simulink model "LevitadorMagnetico_ordenado"  (R2021a)
settings: Solver=ode1  StartTime=0.0  StopTime=1  FixedStep=0.001  RelTol=1e-3
settings Model: Creator=zeta  LastModifiedBy=valen

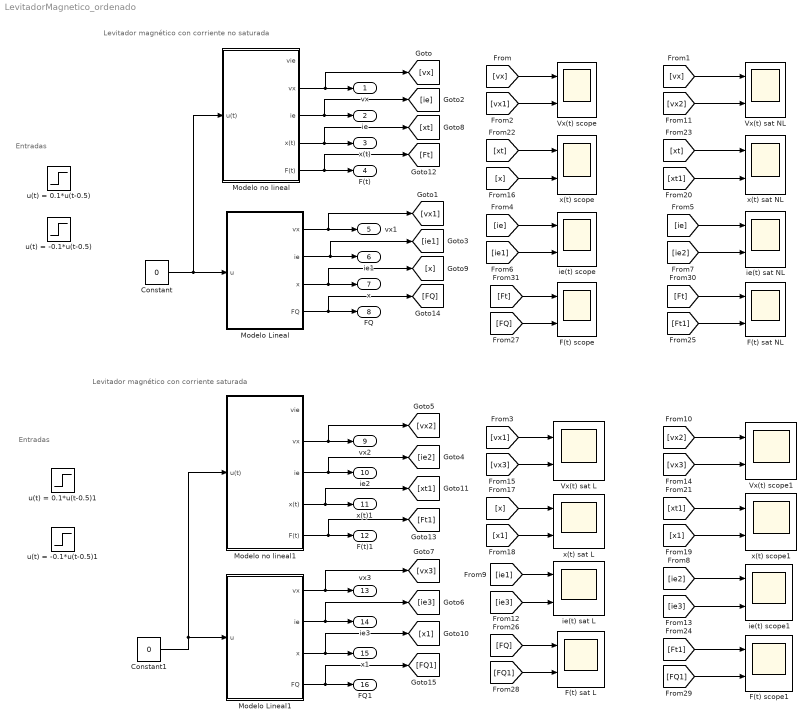
== system LevitadorMagnetico_ordenado ==
  note: Entradas
  note: Levitador magnético con corriente no saturada
  note: Levitador magnético con corriente saturada
  note: Entradas
  Constant : Constant  Value=0
  Constant1 : Constant  Value=0
  F(t) sat L : Scope  NumInputPorts=2
  F(t) sat NL : Scope  NumInputPorts=2
  F(t) scope : Scope  NumInputPorts=2
  F(t) scope1 : Scope  NumInputPorts=2
  Modelo Lineal : Subsystem  mask{Ka=3, Km=1, K1=5888, K2=1536, R=20, L=0.2, uQ=0, xQ=3.2, vxQ=-6.8, ieQ=0, vx_sat_sup=6.8, vx_sat_inf=-10+6.8, x_sat_sup=10-3.2, x_sat_inf=-3.2, m=0.15, g=1000}
      mask prompts: vx_sat_sup "(vx_sat_sup - vxQ)"; vx_sat_inf "(vx_sat_inf- vxQ)"; x_sat_sup "(x_sat_sup - xQ)"; x_sat_inf "(x_sat_inf  - xQ)"
      mask DialogControl Control2 Prompt: Punto de operación:
      mask DialogControl Control3 Prompt: Saturación:
      mask DialogControl Control4 Prompt: otros
  Modelo Lineal1 : Subsystem  mask{Ka=3, Km=1, K1=5888, K2=1536, R=20, L=0.2, uQ=0, xQ=3.2, vxQ=-6.8, ieQ=0, vx_sat_sup=6.8, vx_sat_inf=-10+6.8, x_sat_sup=10-3.2, x_sat_inf=-3.2, m=0.15, g=1000}
      mask prompts: vx_sat_sup "(vx_sat_sup - vxQ)"; vx_sat_inf "(vx_sat_inf- vxQ)"; x_sat_sup "(x_sat_sup - xQ)"; x_sat_inf "(x_sat_inf  - xQ)"
      mask DialogControl Control2 Prompt: Punto de operación:
      mask DialogControl Control3 Prompt: Saturación:
      mask DialogControl Control4 Prompt: otros
  Modelo no lineal : Subsystem
  Modelo no lineal1 : Subsystem
  Vx(t) sat L : Scope  NumInputPorts=2
  Vx(t) sat NL : Scope  NumInputPorts=2
  Vx(t) scope : Scope  NumInputPorts=2
  Vx(t) scope1 : Scope  NumInputPorts=2
  ie(t) sat L : Scope  NumInputPorts=2
  ie(t) sat NL : Scope  NumInputPorts=2
  ie(t) scope : Scope  NumInputPorts=2
  ie(t) scope1 : Scope  NumInputPorts=2
  u(t) = -0.1*u(t-0.5) : Step  Time=0.5  After=-0.1  SampleTime=0
  u(t) = -0.1*u(t-0.5)1 : Step  Time=0.5  After=-0.1  SampleTime=0
  u(t) = 0.1*u(t-0.5) : Step  Time=0.5  After=0.1  SampleTime=0
  u(t) = 0.1*u(t-0.5)1 : Step  Time=0.5  After=0.1  SampleTime=0
  x(t) sat L : Scope  NumInputPorts=2
  x(t) sat NL : Scope  NumInputPorts=2
  x(t) scope : Scope  NumInputPorts=2
  x(t) scope1 : Scope  NumInputPorts=2
  vx : Outport
  ie : Outport  Port=2
  x(t) : Outport  Port=3
  F(t) : Outport  Port=4
  vx1 : Outport  Port=5
  ie1 : Outport  Port=6
  x : Outport  Port=7
  FQ : Outport  Port=8
  vx2 : Outport  Port=9
  ie2 : Outport  Port=10
  x(t)1 : Outport  Port=11
  F(t)1 : Outport  Port=12
  vx3 : Outport  Port=13
  ie3 : Outport  Port=14
  x1 : Outport  Port=15
  FQ1 : Outport  Port=16
  wires:
  Modelo no lineal/2(vx) -> vx/1, [vx]
  Modelo no lineal/4(x(t)) -> x(t)/1, [xt]
  Modelo no lineal/5(F(t)) -> [Ft], F(t)/1
  Modelo Lineal/4(FQ) -> [FQ], FQ/1
  Modelo Lineal/2(ie) -> [ie1], ie1/1
  Modelo Lineal/1(vx) -> vx1/1, [vx1]
  Modelo Lineal/3(x) -> x/1, [x]
  Modelo no lineal/3(ie) -> ie/1, [ie]
  Constant/1 -> Modelo no lineal/1(u(t)), Modelo Lineal/1(u)
  Modelo Lineal1/4(FQ) -> FQ1/1, [FQ1]
  Modelo no lineal1/2(vx) -> vx2/1, [vx2]
  Modelo no lineal1/3(ie) -> ie2/1, [ie2]
  Constant1/1 -> Modelo no lineal1/1(u(t)), Modelo Lineal1/1(u)
  Modelo Lineal1/3(x) -> [x1], x1/1
  Modelo no lineal1/5(F(t)) -> [Ft1], F(t)1/1
  Modelo no lineal1/4(x(t)) -> [xt1], x(t)1/1
  Modelo Lineal1/2(ie) -> ie3/1, [ie3]
  Modelo Lineal1/1(vx) -> vx3/1, [vx3]
  [vx] -> Vx(t) scope/1
  [vx] -> Vx(t) sat NL/1
  [vx1] -> Vx(t) scope/2
  [vx1] -> Vx(t) sat L/1
  [ie] -> ie(t) scope/1
  [ie] -> ie(t) sat NL/1
  [ie1] -> ie(t) scope/2
  [ie1] -> ie(t) sat L/1
  [ie2] -> ie(t) scope1/1
  [ie2] -> ie(t) sat NL/2
  [vx2] -> Vx(t) scope1/1
  [vx2] -> Vx(t) sat NL/2
  [ie3] -> ie(t) sat L/2
  [ie3] -> ie(t) scope1/2
  [vx3] -> Vx(t) scope1/2
  [vx3] -> Vx(t) sat L/2
  [xt] -> x(t) scope/1
  [xt] -> x(t) sat NL/1
  [x] -> x(t) sat L/1
  [x] -> x(t) scope/2
  [xt1] -> x(t) sat NL/2
  [xt1] -> x(t) scope1/1
  [x1] -> x(t) sat L/2
  [x1] -> x(t) scope1/2
  [Ft1] -> F(t) sat NL/2
  [Ft] -> F(t) scope/1
  [Ft] -> F(t) sat NL/1
  [FQ] -> F(t) sat L/1
  [FQ] -> F(t) scope/2
  [Ft1] -> F(t) scope1/1
  [FQ1] -> F(t) scope1/2
  [FQ1] -> F(t) sat L/2

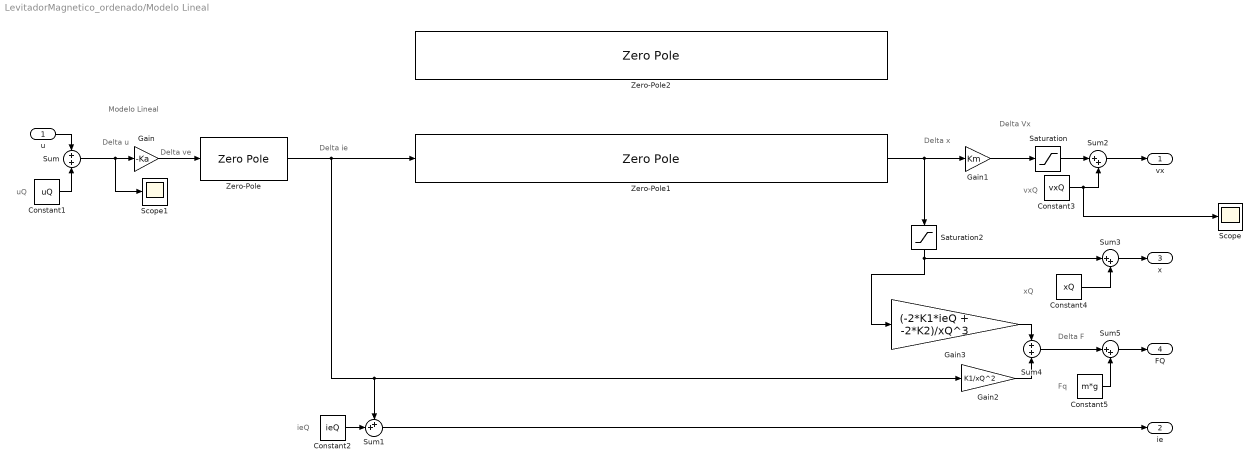
== system LevitadorMagnetico_ordenado/Modelo Lineal ==
  note: Modelo Lineal
  note: Fq
  note: Delta F
  note: vxQ
  note: Delta Vx
  note: Delta x
  note: Delta ie
  note: Delta ve
  note: Delta u
  note: uQ
  note: ieQ
  note: xQ
  u : Inport
  Constant1 : Constant  Value=uQ
  Constant2 : Constant  Value=ieQ
  Constant3 : Constant  Value=vxQ
  Constant4 : Constant  Value=xQ
  Constant5 : Constant  Value=m*g
  Gain : Gain  Gain=-Ka
  Gain1 : Gain  Gain=Km
  Gain2 : Gain  Gain=K1/xQ^2
  Gain3 : Gain  Gain=(-2*K1*ieQ + -2*K2)/xQ^3
  Saturation : Saturate  UpperLimit=vx_sat_sup  LowerLimit=vx_sat_inf
  Saturation2 : Saturate  UpperLimit=x_sat_sup  LowerLimit=x_sat_inf
  Scope : Scope
  Scope1 : Scope
  Sum : Sum  Inputs=+|+
  Sum1 : Sum  Inputs=++|
  Sum2 : Sum  Inputs=|++
  Sum3 : Sum  Inputs=|++
  Sum4 : Sum  Inputs=+|+
  Sum5 : Sum  Inputs=|++
  Zero-Pole : ZeroPole  Zeros=[]  Poles=[-R/L]  Gain=[1/L]
  Zero-Pole1 : ZeroPole  Zeros=[]  Poles=[-25 25]  Gain=[-K1/(m*xQ^2) ]
  Zero-Pole2 : ZeroPole  Zeros=[]  Poles=[-sqrt(2*(K1*ieQ + K2)/(m*xQ^3)) sqrt(2*(K1*ieQ + K2)/(m*xQ^3)) ]  Gain=[-K1/ (m*xQ^2) ]
  vx : Outport
  ie : Outport  Port=2
  x : Outport  Port=3
  FQ : Outport  Port=4
  wires:
  u/1 -> Sum/1
  Sum1/1 -> ie/1
  Sum3/1 -> x/1
  Constant2/1 -> Sum1/2
  Constant4/1 -> Sum3/2
  Sum2/1 -> vx/1
  Sum4/1 -> Sum5/1
  Gain1/1 -> Saturation/1
  Saturation/1 -> Sum2/1
  Constant5/1 -> Sum5/2
  Zero-Pole/1 -> Zero-Pole1/1, Gain2/1, Sum1/1
  Zero-Pole1/1 -> Gain1/1, Saturation2/1
  Sum5/1 -> FQ/1
  Constant1/1 -> Sum/2
  Sum/1 -> Scope1/1, Gain/1
  Gain/1 -> Zero-Pole/1
  Constant3/1 -> Scope/1, Sum2/2
  Gain2/1 -> Sum4/2
  Gain3/1 -> Sum4/1
  Saturation2/1 -> Gain3/1, Sum3/1

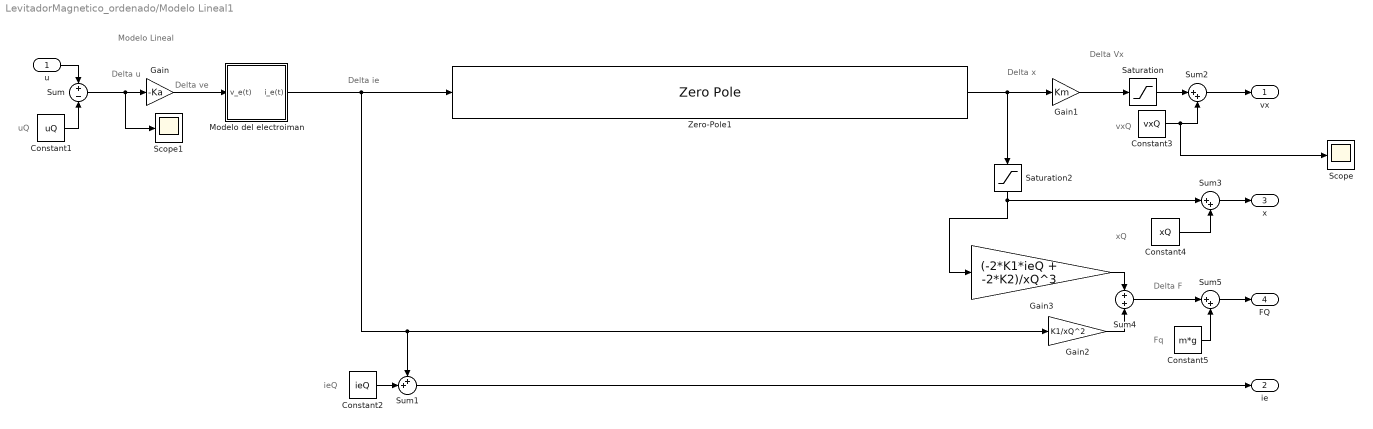
== system LevitadorMagnetico_ordenado/Modelo Lineal1 ==
  note: Modelo Lineal
  note: Fq
  note: Delta F
  note: vxQ
  note: Delta Vx
  note: Delta x
  note: Delta ie
  note: Delta ve
  note: Delta u
  note: uQ
  note: ieQ
  note: xQ
  u : Inport
  Constant1 : Constant  Value=uQ
  Constant2 : Constant  Value=ieQ
  Constant3 : Constant  Value=vxQ
  Constant4 : Constant  Value=xQ
  Constant5 : Constant  Value=m*g
  Gain : Gain  Gain=-Ka
  Gain1 : Gain  Gain=Km
  Gain2 : Gain  Gain=K1/xQ^2
  Gain3 : Gain  Gain=(-2*K1*ieQ + -2*K2)/xQ^3
  Modelo del electroiman : Subsystem  mask{L=0.2, R=20}
      mask prompts: L "L [H]"; R "R [ohm]"
  Saturation : Saturate  UpperLimit=vx_sat_sup  LowerLimit=vx_sat_inf
  Saturation2 : Saturate  UpperLimit=x_sat_sup  LowerLimit=x_sat_inf
  Scope : Scope
  Scope1 : Scope
  Sum : Sum  Inputs=+|-
  Sum1 : Sum  Inputs=++|
  Sum2 : Sum  Inputs=|++
  Sum3 : Sum  Inputs=|++
  Sum4 : Sum  Inputs=+|+
  Sum5 : Sum  Inputs=|++
  Zero-Pole1 : ZeroPole  Zeros=[]  Poles=[-25 25]  Gain=[-K1/(m*xQ^2) ]
  vx : Outport
  ie : Outport  Port=2
  x : Outport  Port=3
  FQ : Outport  Port=4
  wires:
  u/1 -> Sum/1
  Sum1/1 -> ie/1
  Sum3/1 -> x/1
  Constant2/1 -> Sum1/2
  Constant4/1 -> Sum3/2
  Sum2/1 -> vx/1
  Sum4/1 -> Sum5/1
  Gain1/1 -> Saturation/1
  Saturation/1 -> Sum2/1
  Constant5/1 -> Sum5/2
  Modelo del electroiman/1(i_e(t)) -> Zero-Pole1/1, Gain2/1, Sum1/1
  Zero-Pole1/1 -> Gain1/1, Saturation2/1
  Sum5/1 -> FQ/1
  Constant1/1 -> Sum/2
  Sum/1 -> Scope1/1, Gain/1
  Gain/1 -> Modelo del electroiman/1(v_e(t))
  Constant3/1 -> Scope/1, Sum2/2
  Gain2/1 -> Sum4/2
  Gain3/1 -> Sum4/1
  Saturation2/1 -> Gain3/1, Sum3/1

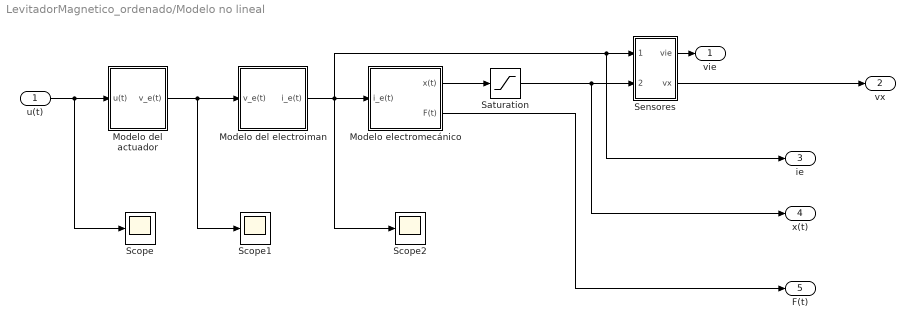
== system LevitadorMagnetico_ordenado/Modelo no lineal ==
  u(t) : Inport
  Modelo del actuador : Subsystem  mask{delta_a=0, K_a=3}
  Modelo del electroiman : Subsystem  mask{L=0.2, R=20}
      mask prompts: L "L [H]"; R "R [ohm]"
  Modelo electromecánico : Subsystem  mask{K_1=5888, K_2=1536, m=0.15, g=1000, x0=3.2, v0=0}
  Saturation : Saturate  UpperLimit=10  LowerLimit=0
  Scope : Scope
  Scope1 : Scope
  Scope2 : Scope
  Sensores : Subsystem  mask{delta_L=0, K_L=20/3, K_m=1, delta_m=10}
  vie : Outport
  vx : Outport  Port=2
  ie : Outport  Port=3
  x(t) : Outport  Port=4
  F(t) : Outport  Port=5
  wires:
  u(t)/1 -> Scope/1, Modelo del actuador/1(u(t))
  Modelo del actuador/1(v_e(t)) -> Scope1/1, Modelo del electroiman/1(v_e(t))
  Sensores/1(vie) -> vie/1
  Modelo del electroiman/1(i_e(t)) -> ie/1, Sensores/1(ie(t)), Modelo electromecánico/1(i_e(t)), Scope2/1
  Modelo electromecánico/1(x(t)) -> Saturation/1
  Modelo electromecánico/2(F(t)) -> F(t)/1
  Sensores/2(vx) -> vx/1
  Saturation/1 -> x(t)/1, Sensores/2(x(t))

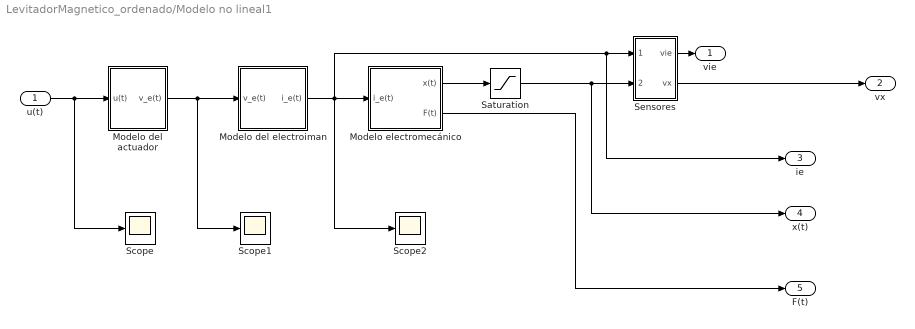
== system LevitadorMagnetico_ordenado/Modelo no lineal1 ==
  u(t) : Inport
  Modelo del actuador : Subsystem  mask{delta_a=0, K_a=3}
  Modelo del electroiman : Subsystem  mask{L=0.2, R=20}
      mask prompts: L "L [H]"; R "R [ohm]"
  Modelo electromecánico : Subsystem  mask{K_1=5888, K_2=1536, m=0.15, g=1000, x0=3.2, v0=0}
  Saturation : Saturate  UpperLimit=10  LowerLimit=0
  Scope : Scope
  Scope1 : Scope
  Scope2 : Scope
  Sensores : Subsystem  mask{delta_L=0, K_L=20/3, K_m=1, delta_m=10}
  vie : Outport
  vx : Outport  Port=2
  ie : Outport  Port=3
  x(t) : Outport  Port=4
  F(t) : Outport  Port=5
  wires:
  u(t)/1 -> Scope/1, Modelo del actuador/1(u(t))
  Modelo del actuador/1(v_e(t)) -> Scope1/1, Modelo del electroiman/1(v_e(t))
  Sensores/1(vie) -> vie/1
  Modelo del electroiman/1(i_e(t)) -> ie/1, Sensores/1(ie(t)), Modelo electromecánico/1(i_e(t)), Scope2/1
  Modelo electromecánico/1(x(t)) -> Saturation/1
  Modelo electromecánico/2(F(t)) -> F(t)/1
  Sensores/2(vx) -> vx/1
  Saturation/1 -> x(t)/1, Sensores/2(x(t))

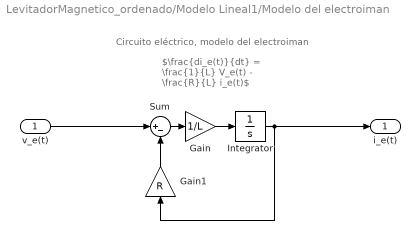
== system LevitadorMagnetico_ordenado/Modelo Lineal1/Modelo del electroiman ==
  note: $\frac{di_e(t)}{dt} = \frac{1}{L} V_e(t) - \frac{R}{L} i_e(t)$
  note: Circuito eléctrico, modelo del electroiman
  v_e(t) : Inport
  Gain : Gain  Gain=1/L
  Gain1 : Gain  Gain=R
  Integrator : Integrator  LimitOutput=on  UpperSaturationLimit=0.01  LowerSaturationLimit=-0.01
  Sum : Sum  Inputs=|+-
  i_e(t) : Outport
  wires:
  v_e(t)/1 -> Sum/1
  Integrator/1 -> i_e(t)/1, Gain1/1
  Gain1/1 -> Sum/2
  Sum/1 -> Gain/1
  Gain/1 -> Integrator/1

== system LevitadorMagnetico_ordenado/Modelo no lineal/Modelo del actuador ==
  note: $v_e(t) = -K_a ~ u(t) + \delta_a$
  note: Modelo del actuador
  u(t) : Inport
  Constant : Constant  Value=delta_a
  Gain : Gain  Gain=K_a
  Sum : Sum  Inputs=+-|
  v_e(t) : Outport
  wires:
  Constant/1 -> Sum/1
  Gain/1 -> Sum/2
  Sum/1 -> v_e(t)/1
  u(t)/1 -> Gain/1

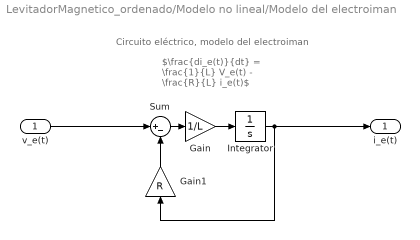
== system LevitadorMagnetico_ordenado/Modelo no lineal/Modelo del electroiman ==
  note: $\frac{di_e(t)}{dt} = \frac{1}{L} V_e(t) - \frac{R}{L} i_e(t)$
  note: Circuito eléctrico, modelo del electroiman
  v_e(t) : Inport
  Gain : Gain  Gain=1/L
  Gain1 : Gain  Gain=R
  Integrator : Integrator
  Sum : Sum  Inputs=|+-
  i_e(t) : Outport
  wires:
  v_e(t)/1 -> Sum/1
  Integrator/1 -> i_e(t)/1, Gain1/1
  Gain1/1 -> Sum/2
  Sum/1 -> Gain/1
  Gain/1 -> Integrator/1

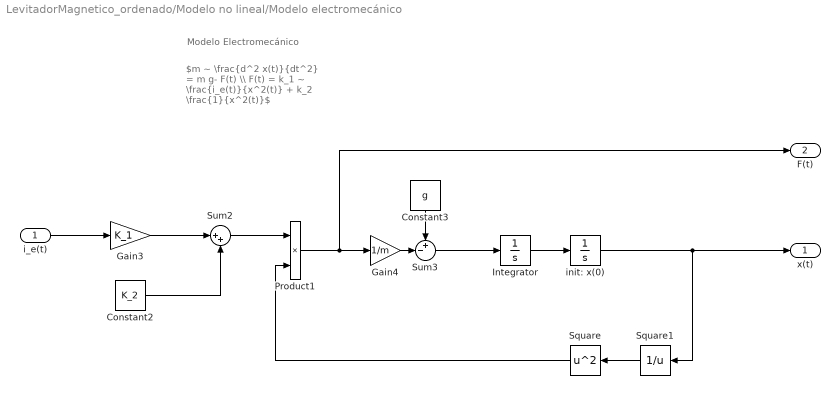
== system LevitadorMagnetico_ordenado/Modelo no lineal/Modelo electromecánico ==
  note: $m ~ \frac{d^2 x(t)}{dt^2} = m g- F(t) \\ F(t) = k_1 ~ \frac{i_e(t)}{x^2(t)} + k_2 \frac{1}{x^2(t)}$
  note: Modelo Electromecánico
  i_e(t) : Inport
  Constant2 : Constant  Value=K_2
  Constant3 : Constant  Value=g
  Gain3 : Gain  Gain=K_1
  Gain4 : Gain  Gain=1/m
  Integrator : Integrator  InitialCondition=v0  LowerSaturationLimit=0
  Product1 : Product
  Square : Math  Operator=square  SaturateOnIntegerOverflow=on
  Square1 : Math  Operator=reciprocal  SaturateOnIntegerOverflow=on
  Sum2 : Sum  Inputs=|++
  Sum3 : Sum  Inputs=+-|
  init: x(0) : Integrator  InitialCondition=x0  UpperSaturationLimit=10  LowerSaturationLimit=1e-10
  x(t) : Outport
  F(t) : Outport  Port=2
  wires:
  i_e(t)/1 -> Gain3/1
  Gain3/1 -> Sum2/1
  Constant2/1 -> Sum2/2
  Sum2/1 -> Product1/1
  Constant3/1 -> Sum3/1
  Gain4/1 -> Sum3/2
  Sum3/1 -> Integrator/1
  Integrator/1 -> init: x(0)/1
  Product1/1 -> F(t)/1, Gain4/1
  Square1/1 -> Square/1
  Square/1 -> Product1/2
  init: x(0)/1 -> x(t)/1, Square1/1

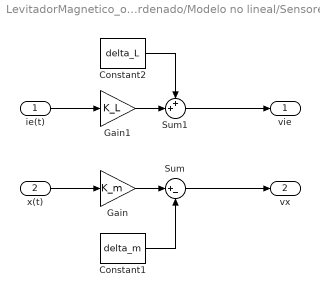
== system LevitadorMagnetico_ordenado/Modelo no lineal/Sensores ==
  ie(t) : Inport
  x(t) : Inport  Port=2
  Constant1 : Constant  Value=delta_m
  Constant2 : Constant  Value=delta_L
  Gain : Gain  Gain=K_m
  Gain1 : Gain  Gain=K_L
  Sum : Sum  Inputs=|+-
  Sum1 : Sum  Inputs=++|
  vie : Outport
  vx : Outport  Port=2
  wires:
  Gain1/1 -> Sum1/2
  Gain/1 -> Sum/1
  Sum1/1 -> vie/1
  Constant2/1 -> Sum1/1
  Sum/1 -> vx/1
  Constant1/1 -> Sum/2
  ie(t)/1 -> Gain1/1
  x(t)/1 -> Gain/1

== system LevitadorMagnetico_ordenado/Modelo no lineal1/Modelo del actuador ==
  note: $v_e(t) = -K_a ~ u(t) + \delta_a$
  note: Modelo del actuador
  u(t) : Inport
  Constant : Constant  Value=delta_a
  Gain : Gain  Gain=K_a
  Sum : Sum  Inputs=+-|
  v_e(t) : Outport
  wires:
  Constant/1 -> Sum/1
  Gain/1 -> Sum/2
  Sum/1 -> v_e(t)/1
  u(t)/1 -> Gain/1

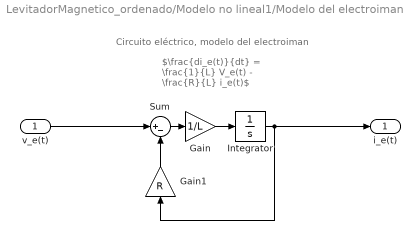
== system LevitadorMagnetico_ordenado/Modelo no lineal1/Modelo del electroiman ==
  note: $\frac{di_e(t)}{dt} = \frac{1}{L} V_e(t) - \frac{R}{L} i_e(t)$
  note: Circuito eléctrico, modelo del electroiman
  v_e(t) : Inport
  Gain : Gain  Gain=1/L
  Gain1 : Gain  Gain=R
  Integrator : Integrator  LimitOutput=on  UpperSaturationLimit=0.01  LowerSaturationLimit=-0.01
  Sum : Sum  Inputs=|+-
  i_e(t) : Outport
  wires:
  v_e(t)/1 -> Sum/1
  Integrator/1 -> i_e(t)/1, Gain1/1
  Gain1/1 -> Sum/2
  Sum/1 -> Gain/1
  Gain/1 -> Integrator/1

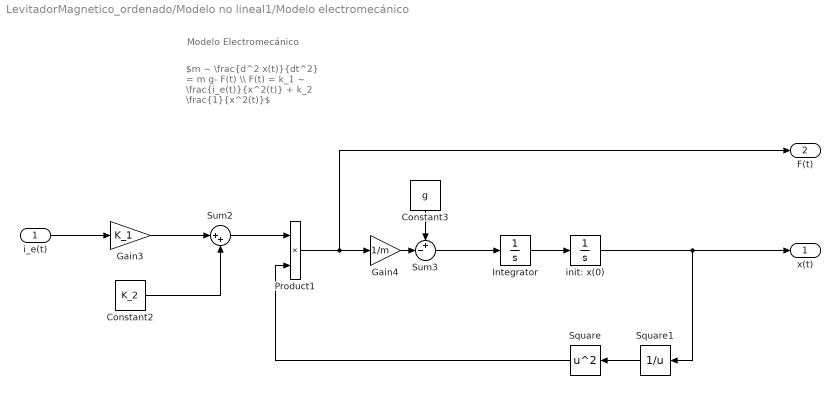
== system LevitadorMagnetico_ordenado/Modelo no lineal1/Modelo electromecánico ==
  note: $m ~ \frac{d^2 x(t)}{dt^2} = m g- F(t) \\ F(t) = k_1 ~ \frac{i_e(t)}{x^2(t)} + k_2 \frac{1}{x^2(t)}$
  note: Modelo Electromecánico
  i_e(t) : Inport
  Constant2 : Constant  Value=K_2
  Constant3 : Constant  Value=g
  Gain3 : Gain  Gain=K_1
  Gain4 : Gain  Gain=1/m
  Integrator : Integrator  InitialCondition=v0  LowerSaturationLimit=0
  Product1 : Product
  Square : Math  Operator=square  SaturateOnIntegerOverflow=on
  Square1 : Math  Operator=reciprocal  SaturateOnIntegerOverflow=on
  Sum2 : Sum  Inputs=|++
  Sum3 : Sum  Inputs=+-|
  init: x(0) : Integrator  InitialCondition=x0  UpperSaturationLimit=10  LowerSaturationLimit=1e-10
  x(t) : Outport
  F(t) : Outport  Port=2
  wires:
  i_e(t)/1 -> Gain3/1
  Gain3/1 -> Sum2/1
  Constant2/1 -> Sum2/2
  Sum2/1 -> Product1/1
  Constant3/1 -> Sum3/1
  Gain4/1 -> Sum3/2
  Sum3/1 -> Integrator/1
  Integrator/1 -> init: x(0)/1
  Product1/1 -> F(t)/1, Gain4/1
  Square1/1 -> Square/1
  Square/1 -> Product1/2
  init: x(0)/1 -> x(t)/1, Square1/1

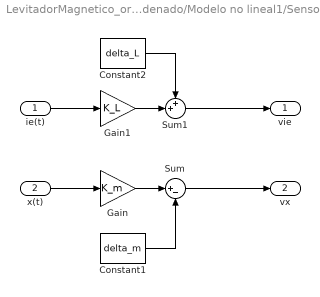
== system LevitadorMagnetico_ordenado/Modelo no lineal1/Sensores ==
  ie(t) : Inport
  x(t) : Inport  Port=2
  Constant1 : Constant  Value=delta_m
  Constant2 : Constant  Value=delta_L
  Gain : Gain  Gain=K_m
  Gain1 : Gain  Gain=K_L
  Sum : Sum  Inputs=|+-
  Sum1 : Sum  Inputs=++|
  vie : Outport
  vx : Outport  Port=2
  wires:
  Gain1/1 -> Sum1/2
  Gain/1 -> Sum/1
  Sum1/1 -> vie/1
  Constant2/1 -> Sum1/1
  Sum/1 -> vx/1
  Constant1/1 -> Sum/2
  ie(t)/1 -> Gain1/1
  x(t)/1 -> Gain/1
